simulink library "controller_lib"  (R2017b)
settings: Solver=VariableStepAuto  StartTime=0.0  StopTime=10.0  RelTol=1e-3
libraries: simulink x1
settings Model: Creator=Máté  LastModifiedBy=Máté

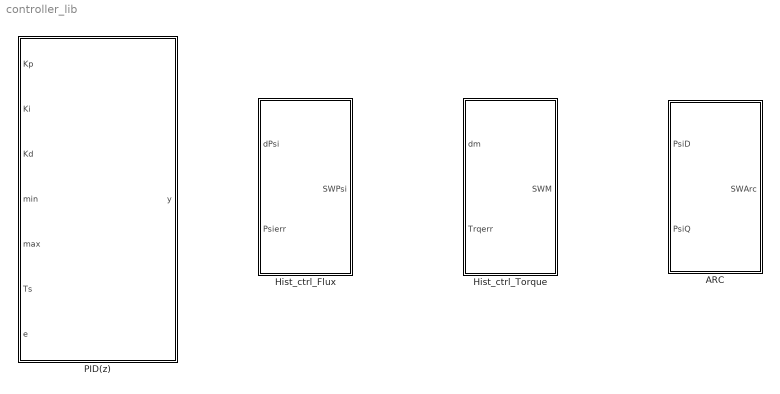
== system controller_lib ==
  ARC : Subsystem
  Hist_ctrl_Flux : Subsystem
  Hist_ctrl_Torque : Subsystem
  PID(z) : Subsystem

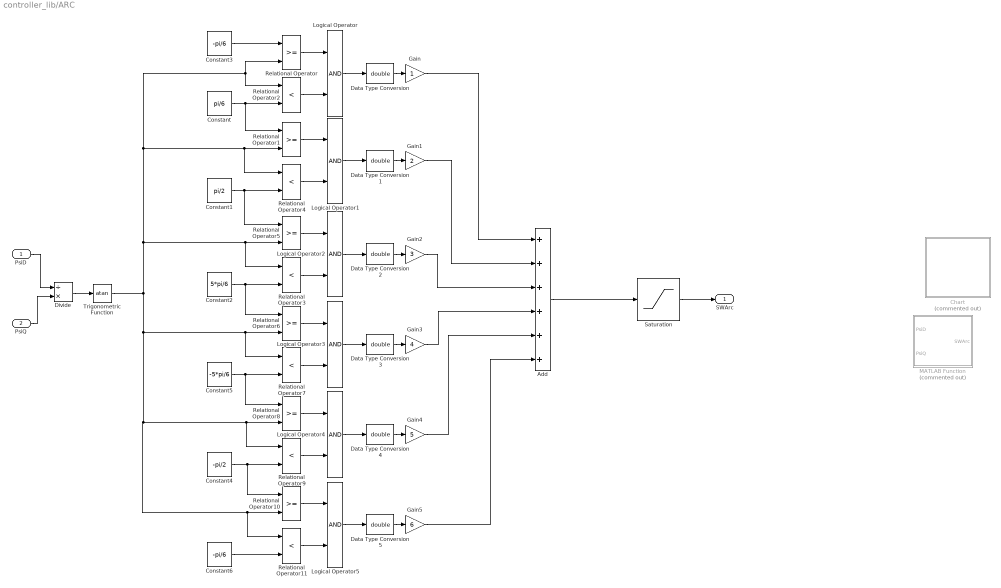
== system controller_lib/ARC ==
  PsiD : Inport
  PsiQ : Inport  Port=2
  Add : Sum  Inputs=++++++
  Chart : Stateflow chart  Commented=on  TreatAsAtomicUnit=on
  Constant : Constant  Value=pi/6  VectorParams1D=off  SampleTime=-1
  Constant1 : Constant  Value=pi/2  VectorParams1D=off  SampleTime=-1
  Constant2 : Constant  Value=5*pi/6  VectorParams1D=off  SampleTime=-1
  Constant3 : Constant  Value=-pi/6  VectorParams1D=off  SampleTime=-1
  Constant4 : Constant  Value=-pi/2  VectorParams1D=off  SampleTime=-1
  Constant5 : Constant  Value=-5*pi/6  VectorParams1D=off  SampleTime=-1
  Constant6 : Constant  Value=-pi/6  VectorParams1D=off  SampleTime=-1
  Data Type Conversion{,1..5} (6 alike) : DataTypeConversion  OutDataTypeStr=double
  Divide : Product  Inputs=/*
  Gain : Gain
  Gain1 : Gain  Gain=2
  Gain2 : Gain  Gain=3
  Gain3 : Gain  Gain=4
  Gain4 : Gain  Gain=5
  Gain5 : Gain  Gain=6
  Logical Operator{,1..5} (6 alike) : Logic  AllPortsSameDT=off  OutDataTypeStr=boolean
  MATLAB Function : MATLAB Function  Commented=on  TreatAsAtomicUnit=on
  Relational Operator{,1,5..6,8,10} (6 alike) : RelationalOperator  OutDataTypeStr=boolean  RndMeth=Simplest
  Relational Operator{2..4,7,9,11} (6 alike) : RelationalOperator  Operator=<  OutDataTypeStr=boolean  RndMeth=Simplest
  Saturation : Saturate  UpperLimit=6  LowerLimit=1
  Trigonometric Function : Trigonometry  Operator=atan
  SWArc : Outport
  wires:
  Constant3/1 -> Relational Operator/1
  Trigonometric Function/1 -> Relational Operator11/1, Relational Operator10/2, Relational Operator9/1, Relational Operator8/2, Relational Operator7/1, Relational Operator6/2, Relational Operator3/1, Relational Operator5/2, Relational Operator4/1, Relational Operator1/2, Relational Operator/2, Relational Operator2/1
  Constant/1 -> Relational Operator1/1, Relational Operator2/2
  Constant1/1 -> Relational Operator5/1, Relational Operator4/2
  Constant2/1 -> Relational Operator6/1, Relational Operator3/2
  Constant5/1 -> Relational Operator8/1, Relational Operator7/2
  Constant4/1 -> Relational Operator10/1, Relational Operator9/2
  Constant6/1 -> Relational Operator11/2
  Relational Operator/1 -> Logical Operator/1
  Relational Operator2/1 -> Logical Operator/2
  Relational Operator1/1 -> Logical Operator1/1
  Relational Operator4/1 -> Logical Operator1/2
  Relational Operator5/1 -> Logical Operator2/1
  Relational Operator3/1 -> Logical Operator2/2
  Relational Operator6/1 -> Logical Operator3/1
  Relational Operator7/1 -> Logical Operator3/2
  Relational Operator8/1 -> Logical Operator4/1
  Relational Operator9/1 -> Logical Operator4/2
  Relational Operator10/1 -> Logical Operator5/1
  Relational Operator11/1 -> Logical Operator5/2
  Gain/1 -> Add/1
  Gain1/1 -> Add/2
  Gain2/1 -> Add/3
  Gain3/1 -> Add/4
  Gain4/1 -> Add/5
  Gain5/1 -> Add/6
  Saturation/1 -> SWArc/1
  Logical Operator/1 -> Data Type Conversion/1
  Data Type Conversion/1 -> Gain/1
  Logical Operator1/1 -> Data Type Conversion1/1
  Data Type Conversion1/1 -> Gain1/1
  Logical Operator2/1 -> Data Type Conversion2/1
  Data Type Conversion2/1 -> Gain2/1
  Logical Operator3/1 -> Data Type Conversion3/1
  Data Type Conversion3/1 -> Gain3/1
  Logical Operator4/1 -> Data Type Conversion4/1
  Data Type Conversion4/1 -> Gain4/1
  Logical Operator5/1 -> Data Type Conversion5/1
  Data Type Conversion5/1 -> Gain5/1
  Add/1 -> Saturation/1
  PsiQ/1 -> Divide/2
  Divide/1 -> Trigonometric Function/1
  PsiD/1 -> Divide/1

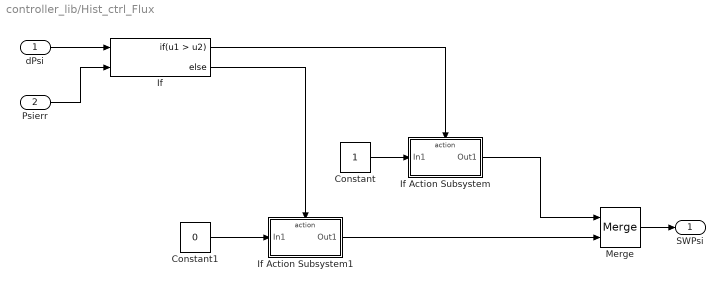
== system controller_lib/Hist_ctrl_Flux ==
  dPsi : Inport
  Psierr : Inport  Port=2
  Constant : Constant
  Constant1 : Constant  Value=0
  If : If  NumInputs=2  IfExpression=u1 > u2
  If Action Subsystem : Subsystem  TreatAsAtomicUnit=on
  If Action Subsystem1 : Subsystem  TreatAsAtomicUnit=on
  Merge : Merge
  SWPsi : Outport
  wires:
  Psierr/1 -> If/2
  dPsi/1 -> If/1
  If/1 -> If Action Subsystem/Action
  Constant/1 -> If Action Subsystem/1(In1)
  If/2 -> If Action Subsystem1/Action
  Constant1/1 -> If Action Subsystem1/1(In1)
  Merge/1 -> SWPsi/1
  If Action Subsystem/1(Out1) -> Merge/1
  If Action Subsystem1/1(Out1) -> Merge/2

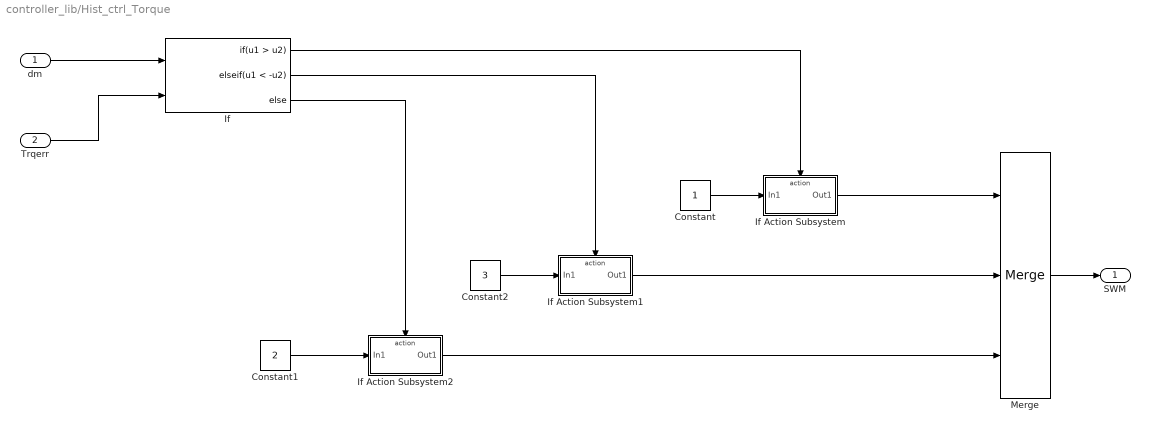
== system controller_lib/Hist_ctrl_Torque ==
  dm : Inport
  Trqerr : Inport  Port=2
  Constant : Constant
  Constant1 : Constant  Value=2
  Constant2 : Constant  Value=3
  If : If  NumInputs=2  IfExpression=u1 > u2  ElseIfExpressions=u1 < -u2
  If Action Subsystem : Subsystem  TreatAsAtomicUnit=on
  If Action Subsystem1 : Subsystem  TreatAsAtomicUnit=on
  If Action Subsystem2 : Subsystem  TreatAsAtomicUnit=on
  Merge : Merge  Inputs=3
  SWM : Outport
  wires:
  dm/1 -> If/1
  If/1 -> If Action Subsystem/Action
  If/2 -> If Action Subsystem1/Action
  If/3 -> If Action Subsystem2/Action
  Constant/1 -> If Action Subsystem/1(In1)
  Constant1/1 -> If Action Subsystem2/1(In1)
  Constant2/1 -> If Action Subsystem1/1(In1)
  Merge/1 -> SWM/1
  If Action Subsystem/1(Out1) -> Merge/1
  If Action Subsystem1/1(Out1) -> Merge/2
  If Action Subsystem2/1(Out1) -> Merge/3
  Trqerr/1 -> If/2

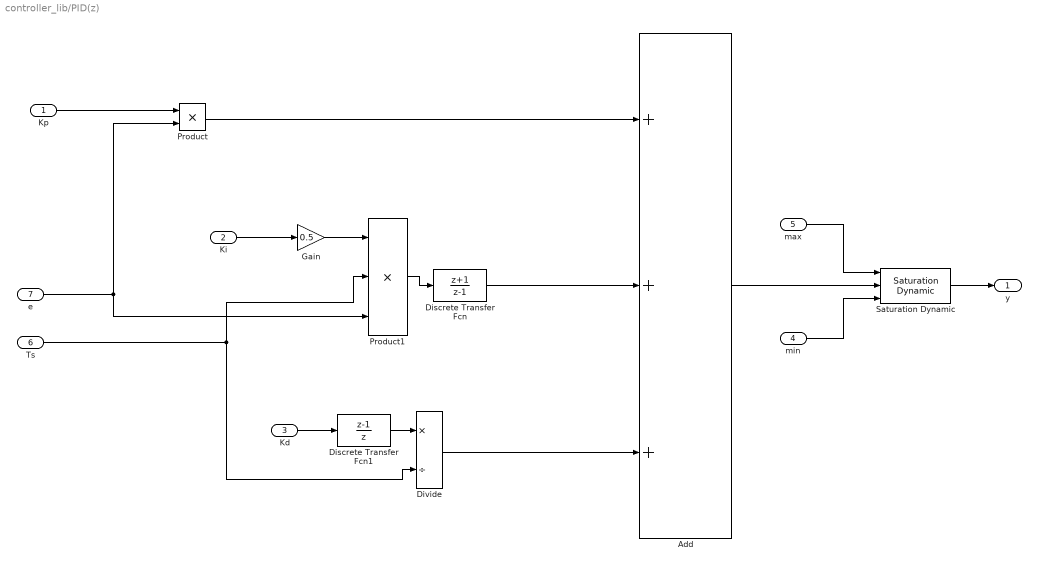
== system controller_lib/PID(z) ==
  Kp : Inport
  Ki : Inport  Port=2
  Kd : Inport  Port=3
  min : Inport  Port=4
  "max " : Inport  Port=5
  Ts : Inport  Port=6
  e : Inport  Port=7
  Add : Sum  Inputs=+++
  Discrete Transfer Fcn : DiscreteTransferFcn  Numerator=[1 1]  Denominator=[1 -1]
  Discrete Transfer Fcn1 : DiscreteTransferFcn  Numerator=[1 -1]  Denominator=[1 0]
  Divide : Product  Inputs=*/
  Gain : Gain  Gain=0.5
  Product : Product
  Product1 : Product  Inputs=3
  Saturation Dynamic : simulink/Discontinuities/Saturation Dynamic  OutMin=[]  OutMax=[]  OutDataTypeStr=Inherit: Same as second input  OutDataType=fixdt(1, 16)  OutScaling=2^-10  DoSatur=off
  y : Outport
  wires:
  min/1 -> Saturation Dynamic/3
  "max "/1 -> Saturation Dynamic/1
  Saturation Dynamic/1 -> y/1
  Add/1 -> Saturation Dynamic/2
  e/1 -> Product/2, Product1/3
  Kp/1 -> Product/1
  Ki/1 -> Gain/1
  Gain/1 -> Product1/1
  Product1/1 -> Discrete Transfer Fcn/1
  Ts/1 -> Divide/2, Product1/2
  Discrete Transfer Fcn1/1 -> Divide/1
  Kd/1 -> Discrete Transfer Fcn1/1
  Product/1 -> Add/1
  Discrete Transfer Fcn/1 -> Add/2
  Divide/1 -> Add/3

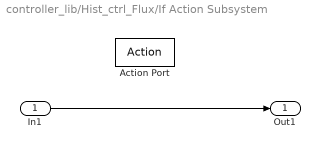
== system controller_lib/Hist_ctrl_Flux/If Action Subsystem ==
  In1 : Inport
  Action Port : ActionPort
  Out1 : Outport
  wires:
  In1/1 -> Out1/1

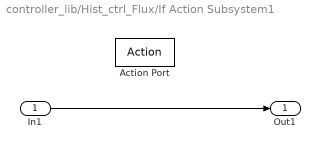
== system controller_lib/Hist_ctrl_Flux/If Action Subsystem1 ==
  In1 : Inport
  Action Port : ActionPort
  Out1 : Outport
  wires:
  In1/1 -> Out1/1

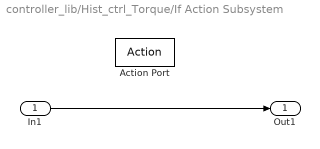
== system controller_lib/Hist_ctrl_Torque/If Action Subsystem ==
  In1 : Inport
  Action Port : ActionPort  ActionType=then
  Out1 : Outport
  wires:
  In1/1 -> Out1/1

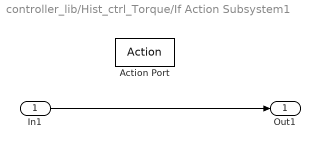
== system controller_lib/Hist_ctrl_Torque/If Action Subsystem1 ==
  In1 : Inport
  Action Port : ActionPort  ActionType=elseif
  Out1 : Outport
  wires:
  In1/1 -> Out1/1

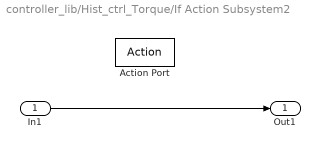
== system controller_lib/Hist_ctrl_Torque/If Action Subsystem2 ==
  In1 : Inport
  Action Port : ActionPort  ActionType=else
  Out1 : Outport
  wires:
  In1/1 -> Out1/1

== matlab function controller_lib/ARC/MATLAB Function ==
  data: PsiD input; SWArc output; PsiQ input
function SWArc = arc_function(PsiD,PsiQ)

angle = atan(PsiQ/PsiD);
double x;
    
if (11*pi/6 < angle) && (angle <= pi/6)
        x = 1; 
        
        elseif (pi/6 < angle) && (angle <= pi/2)
            x = 2;
               
            elseif (pi/2 < angle) && (angle <= 5*pi/6)
                 x = 3;
                    
                 elseif (5*pi/6 < angle) && (angle <= 7*pi/6)
                       x = 4;
                            
                        elseif (7*pi/6 < angle) && (angle <= 3*pi/2)
                                x = 5;
    else 
        x = 6;
end

SWArc = x;

== stateflow chart controller_lib/ARC/Chart ==
  (junction 1) -> (junction 2) [order 4] : [x <= 30 && x > -30]{y = 1}
  (junction 1) -> (junction 6) [order 5] : [x <= 90 && x > 30]{y = 2}
  (junction 1) -> (junction 16) [order 2] : [x <= 330 && x > 270]{y = 6}
  (junction 23) -> (junction 1)
  (junction 1) -> (junction 4) [order 6] : [x <= 150 && x > 90]{y = 3}
  (junction 1) -> (junction 13) [order 3] : [x <= 270 && x > 210]{y = 5}
  (junction 1) -> (junction 8) [order 1] : [x <= 210 && x > 150]{y = 4}
